simulink model "eg"  (R2019a)
settings: Solver=FixedStepDiscrete  StartTime=0.0  StopTime=Inf  FixedStep=0.0001  RelTol=1e-3
libraries: simulink x2
settings Model: Creator=User  LastModifiedBy=User

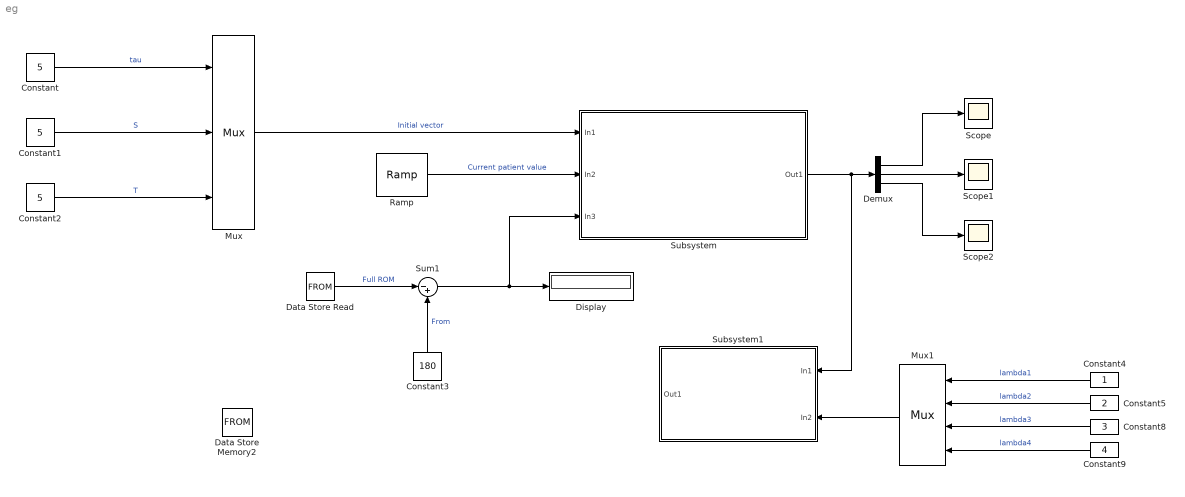
== system eg ==
  Constant : Constant  Value=5
  Constant1 : Constant  Value=5
  Constant2 : Constant  Value=5
  Constant3 : Constant  Value=180
  Constant4 : Constant
  Constant5 : Constant  Value=2
  Constant8 : Constant  Value=3
  Constant9 : Constant  Value=4
  Data Store Memory2 : DataStoreMemory  DataStoreName=FROM  ReadBeforeWriteMsg=warning  WriteAfterWriteMsg=warning  WriteAfterReadMsg=warning  ShowAdditionalParam=off
  Data Store Read : DataStoreRead  DataStoreName=FROM
  Demux : Demux  Outputs=3
  Display : Display
  Mux : Mux  Inputs=3
      settings: DisplayOption=signals
  Mux1 : Mux
      settings: DisplayOption=signals
  Ramp : simulink/Sources/Ramp  slope=5  start=0  InitialOutput=0
  Scope : Scope
  Scope1 : Scope
  Scope2 : Scope
  Subsystem : Subsystem
  Subsystem1 : Subsystem
  Sum1 : Sum  Inputs=|-+
  wires:
  Constant/1 -> Mux/1  "tau"
  Constant1/1 -> Mux/2  "S"
  Constant2/1 -> Mux/3  "T"
  Mux/1 -> Subsystem/1(In1)  "Initial vector"
  Ramp/1 -> Subsystem/2(In2)  "Current patient value"
  Subsystem/1(Out1) -> Subsystem1/1(In1), Demux/1
  Demux/1 -> Scope/1
  Demux/2 -> Scope1/1
  Demux/3 -> Scope2/1
  Mux1/1 -> Subsystem1/2(In2)
  Constant4/1 -> Mux1/1  "lambda1"
  Constant5/1 -> Mux1/2  "lambda2"
  Constant8/1 -> Mux1/3  "lambda3"
  Constant9/1 -> Mux1/4  "lambda4"
  Sum1/1 -> Display/1, Subsystem/3(In3)
  Constant3/1 -> Sum1/2  "From"
  Data Store Read/1 -> Sum1/1  "Full ROM"

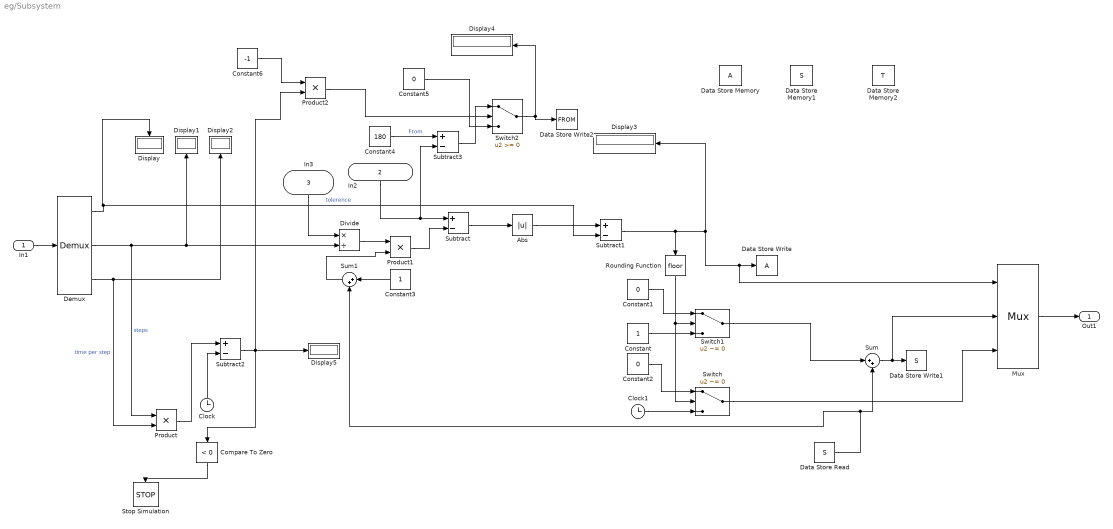
== system eg/Subsystem ==
  In1 : Inport
  In2 : Inport  Port=2
  In3 : Inport  Port=3
  Abs : Abs
  Clock : Clock
  Clock1 : Clock
  Compare To Zero : simulink/Logic and Bit Operations/Compare To Zero  relop=<  OutDataTypeStr=boolean
  Constant : Constant
  Constant1 : Constant  Value=0
  Constant2 : Constant  Value=0
  Constant3 : Constant
  Constant4 : Constant  Value=180
  Constant5 : Constant  Value=0
  Constant6 : Constant  Value=-1
  Data Store Memory : DataStoreMemory  ReadBeforeWriteMsg=warning  WriteAfterWriteMsg=warning  WriteAfterReadMsg=warning  ShowAdditionalParam=off
  Data Store Memory1 : DataStoreMemory  DataStoreName=S  ReadBeforeWriteMsg=warning  WriteAfterWriteMsg=warning  WriteAfterReadMsg=warning  ShowAdditionalParam=off
  Data Store Memory2 : DataStoreMemory  DataStoreName=T  ReadBeforeWriteMsg=warning  WriteAfterWriteMsg=warning  WriteAfterReadMsg=warning  ShowAdditionalParam=off
  Data Store Read : DataStoreRead  DataStoreName=S
  Data Store Write : DataStoreWrite
  Data Store Write1 : DataStoreWrite  DataStoreName=S
  Data Store Write2 : DataStoreWrite  DataStoreName=FROM
  Demux : Demux  Outputs=3
  Display{,1..5} (6 alike) : Display
      settings: Decimation=3
  Divide : Product  Inputs=*/
  Mux : Mux  Inputs=3
      settings: DisplayOption=signals
  Product : Product
  Product1 : Product
  Product2 : Product
  Rounding Function : Rounding
  Stop Simulation : Stop
  Subtract{,1..3} (4 alike) : Sum  Inputs=+-
  Sum : Sum  Inputs=|++
  Sum1 : Sum  Inputs=|++
  Switch : Switch  Criteria=u2 ~= 0
  Switch1 : Switch  Criteria=u2 ~= 0
  Switch2 : Switch
  Out1 : Outport
  wires:
  In1/1 -> Demux/1
  Demux/1 -> Subtract1/2, Display/1  "tolerence"
  Demux/3 -> Product/2, Display2/1  "time per step"
  Demux/2 -> Product/1, Divide/2, Display1/1  "steps"
  In3/1 -> Divide/1
  In2/1 -> Subtract3/2, Subtract/1
  Subtract/1 -> Abs/1
  Abs/1 -> Subtract1/1
  Clock/1 -> Subtract2/2
  Subtract2/1 -> Product2/2, Display5/1, Compare To Zero/1
  Compare To Zero/1 -> Stop Simulation/1
  Mux/1 -> Out1/1
  Sum/1 -> Mux/2, Data Store Write1/1
  Switch1/1 -> Sum/1
  Data Store Read/1 -> Sum/2, Sum1/2
  Clock1/1 -> Switch/3
  Switch/1 -> Mux/3
  Subtract1/1 -> Rounding Function/1, Mux/1, Data Store Write/1, Display3/1
  Constant/1 -> Switch1/3
  Constant1/1 -> Switch1/1
  Constant2/1 -> Switch/1
  Product/1 -> Subtract2/1
  Divide/1 -> Product1/1
  Sum1/1 -> Product1/2
  Constant3/1 -> Sum1/1
  Product1/1 -> Subtract/2
  Rounding Function/1 -> Switch1/2, Switch/2
  Constant4/1 -> Subtract3/1  "From"
  Subtract3/1 -> Switch2/1
  Switch2/1 -> Data Store Write2/1, Display4/1
  Constant5/1 -> Switch2/3
  Constant6/1 -> Product2/1
  Product2/1 -> Switch2/2

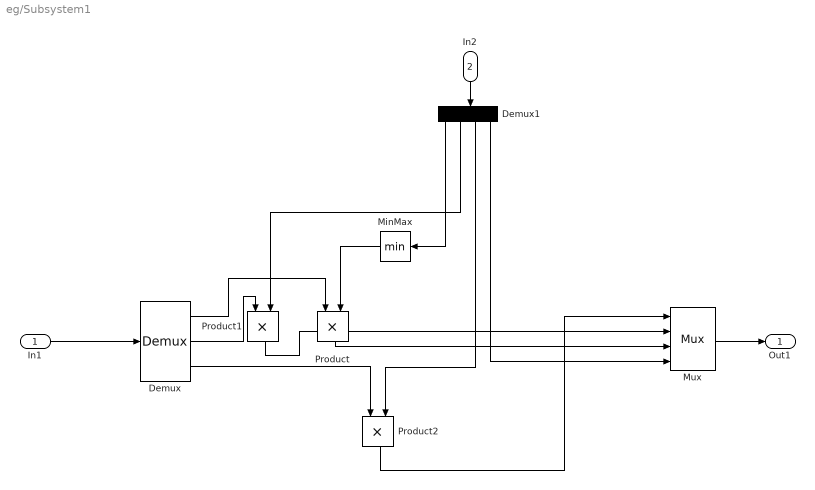
== system eg/Subsystem1 ==
  In1 : Inport
  In2 : Inport  Port=2
  Demux : Demux  Outputs=3
  Demux1 : Demux
  MinMax : MinMax
  Mux : Mux
      settings: DisplayOption=signals
  Product : Product
  Product1 : Product
  Product2 : Product
  Out1 : Outport
  wires:
  In1/1 -> Demux/1
  In2/1 -> Demux1/1
  Demux/1 -> Product/1
  Demux/2 -> Product1/1
  Demux1/2 -> Product1/2
  Demux/3 -> Product2/1
  Demux1/3 -> Product2/2
  Mux/1 -> Out1/1
  Product2/1 -> Mux/1
  Product1/1 -> Mux/2
  Product/1 -> Mux/3
  Demux1/4 -> Mux/4
  Demux1/1 -> MinMax/1
  MinMax/1 -> Product/2
